simulink model "test_friction_lut"  (R2022b)
settings: Solver=ode4  StartTime=0.0  StopTime=100.0  FixedStep=1e-3  RelTol=1e-3
values from neighbouring files (symbols this model uses):
  BuildingHeight = 10    [test_LUT_friction.m]
  LUT_Coloumb_friction = 10./( (LUT_position-3).^2+1)    [test_LUT_friction.m]
  LUT_position = linspace(0,BuildingHeight,10)'    [test_LUT_friction.m]
  LUT_viscous_friction = (0.1+0.05./BuildingHeight*LUT_position).*ones(length(LUT_position),1)    [test_LUT_friction.m]
libraries: simulink x1, LumpedParameterLiftModels x1
settings Model: Creator=manue  LastModifiedBy=manue

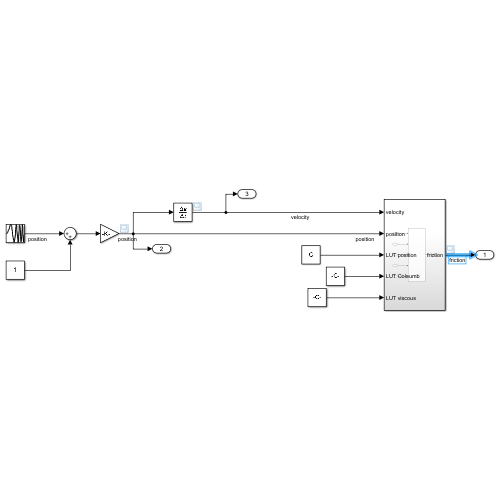
[thumbnail: Simulink's stored preview of the top-level diagram]
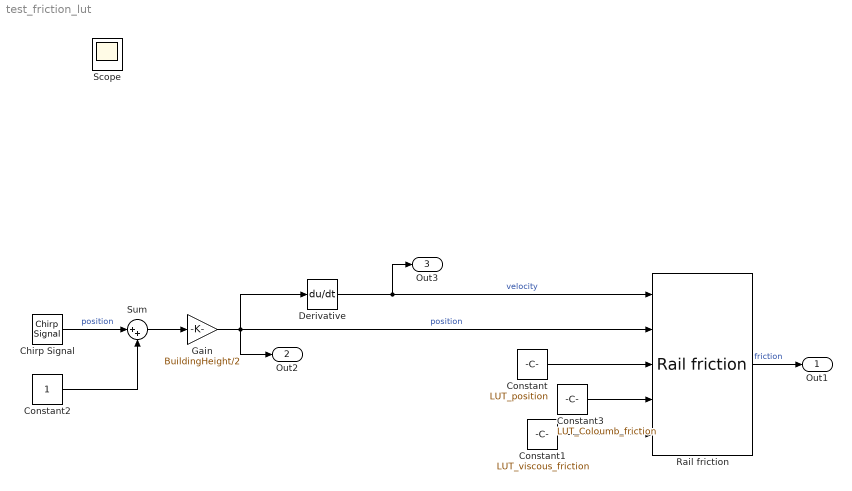
== system test_friction_lut ==
  Chirp Signal : simulink/Sources/Chirp Signal  f1=0.1  T=100  f2=1
  Constant : Constant  Value=LUT_position
  Constant1 : Constant  Value=LUT_viscous_friction
  Constant2 : Constant
  Constant3 : Constant  Value=LUT_Coloumb_friction
  Derivative : Derivative
  Gain : Gain  Gain=BuildingHeight/2
  Rail friction : LumpedParameterLiftModels/Rail friction  SystemSampleTime=-1  VariantActivationTime=update diagram  Latency=0  AutoFrameSizeCalculation=off
  Sum : Sum  Inputs=|++
  Out1 : Outport
  Out2 : Outport  Port=2
  Out3 : Outport  Port=3
  Scope : Scope
  wires:
  Sum/1 -> Gain/1
  Derivative/1 -> Out3/1, Rail friction/1  "velocity"
  Constant/1 -> Rail friction/3
  Constant3/1 -> Rail friction/4
  Constant1/1 -> Rail friction/5
  Rail friction/1 -> Out1/1  "friction"
  Gain/1 -> Out2/1, Rail friction/2, Derivative/1  "position"
  Chirp Signal/1 -> Sum/1  "position"
  Constant2/1 -> Sum/2
